simulink model "simp"  (R2012b)
settings: Solver=ode45  StartTime=0.0  StopTime=1000  FixedStep=0.01  RelTol=1e-3
values from neighbouring files (symbols this model uses):
  A43 = gama / Jp - (L * gama) / (Jp * beta)    (= 8.61159929701)    [para.m]    (also in test.m = 8.13653136531)
  B4 = (L / beta - 1) / Jp    (= -0.00439367311072)    [para.m]    (also in test.m = -0.00615006150062)
  f4 = 100    [para.m]
  gama1 = -4    [para.m]
  gama2 = -10000    [para.m]
  K2max = 100    [para.m]
  Kd0 = 2 * ksi * wn / B4    (= -3218.264)    [para.m]
  Kp0 = (wn ^ 2 + A43) / B4    (= -24720)    [para.m]
  ksi = 0.707    [para.m]
  Kthi0 = 1000    [para.m]
  p11 = ksi / wn + (wn ^ 2 + 1) / (4 * ksi)    (= 35.7849857143)    [para.m]
  p12 = 1 / (2 * wn ^ 2)    (= 0.005)    [para.m]
  p22 = (wn ^ 2 + 1) / (4 * ksi * wn ^ 3)    (= 0.0357142857143)    [para.m]
  wn = 10    [para.m]
settings Model: Creator=Administrator  LastModifiedBy=Administrator
settings DebuggingCC: MaxConsecutiveZCsMsg=warning

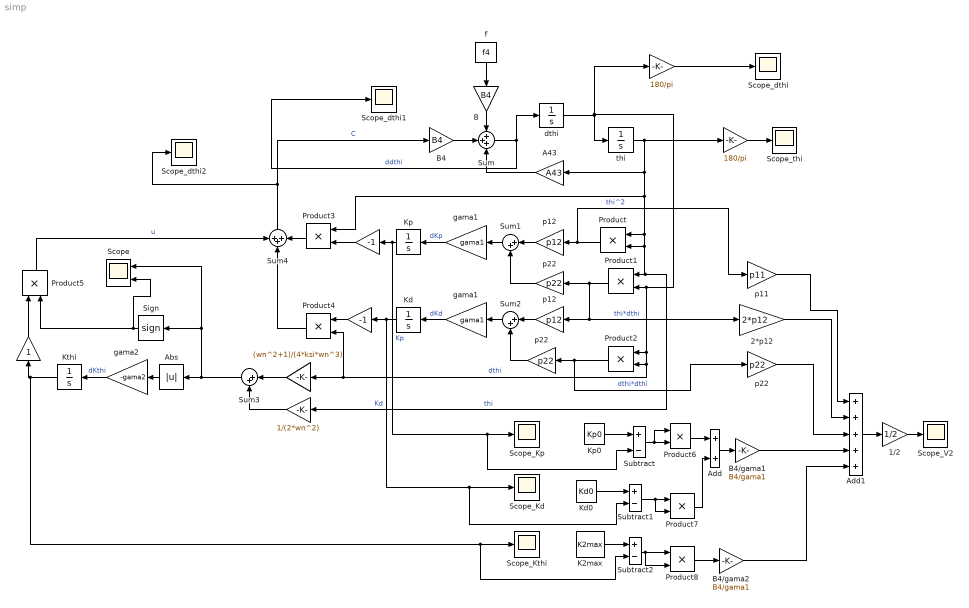
== system simp ==
  "    " : Gain  Gain=180/pi
  "         " : Gain  Gain=(wn^2+1)/(4*ksi*wn^3)
  "          " : Gain  Gain=1/(2*wn^2)
  "            " : Gain  Gain=-1
  "             " : Gain  Gain=180/pi
  "              " : Gain  Gain=-1
  "               " : Gain
  "  p11" : Gain  Gain=p11
  "  p12 " : Gain  Gain=p12
  " 2*p12" : Gain  Gain=2*p12
  1/2 : Gain  Gain=1/2
  A43 : Gain  Gain=A43
  Abs : Abs
  Add : Sum
  Add1 : Sum  Inputs=+++++
  B : Gain  Gain=B4
  B4 : Gain  Gain=B4
  B4/gama1 : Gain  Gain=B4/gama1
  B4/gama2 : Gain  Gain=B4/gama1
  K2max : Constant  Value=K2max
  Kd : Integrator  InitialCondition=Kd0
  Kd0 : Constant  Value=Kd0
  Kp : Integrator  InitialCondition=Kp0
  Kp0 : Constant  Value=Kp0
  Kthi : Integrator  InitialCondition=Kthi0
  Product{,1..8} (9 alike) : Product  RndMeth=Zero
  Scope : Scope  NumInputPorts=2
      settings: YMin=-5~-5  YMax=5~5  SaveName=ScopeData5
  Scope_Kd : Scope
      settings: SaveName=ScopeData3
  Scope_Kp : Scope
      settings: SaveName=ScopeData2
  Scope_Kthi : Scope
      settings: SaveName=ScopeData4
  Scope_V2 : Scope
      settings: SaveName=ScopeData6
  Scope_dthi : Scope
  Scope_dthi1 : Scope
      settings: SaveName=ScopeData7
  Scope_dthi2 : Scope
      settings: SaveName=ScopeData8
  Scope_thi : Scope
  Sign : Signum  ZeroCross=off
  Subtract : Sum  Inputs=+-
  Subtract1 : Sum  Inputs=+-
  Subtract2 : Sum  Inputs=+-
  Sum : Sum  Inputs=+++
  Sum1 : Sum  Inputs=|++
  Sum2 : Sum  Inputs=|++
  Sum3 : Sum  Inputs=|++
  Sum4 : Sum  Inputs=+++
  dthi : Integrator
  f : Constant  Value=f4
  gama1 : Gain  Gain=gama1
  "gama1      " : Gain  Gain=gama1
  gama2 : Gain  Gain=-gama2
  p12 : Gain  Gain=p12
  p22 : Gain  Gain=p22
  "p22 " : Gain  Gain=p22
  "p22  " : Gain  Gain=p22
  thi : Integrator  InitialCondition=15*pi/180
  wires:
  dthi/1 -> thi/1, Product4/2, "         "/1, Product2/2, Product2/1, Product1/2, "    "/1  "dthi"
  thi/1 -> "             "/1, Product1/1, "          "/1, Product/2, Product/1, Product3/1, A43/1  "thi"
  B4/1 -> Sum/2
  f/1 -> B/1
  A43/1 -> Sum/3
  Sum/1 -> dthi/1, Scope_dthi1/1  "ddthi"
  Product/1 -> "  p11"/1, p12/1  "thi^2"
  Product1/1 -> p22/1, " 2*p12"/1, "  p12 "/1  "thi*dthi"
  p12/1 -> Sum1/1
  p22/1 -> Sum1/2
  Product2/1 -> "p22 "/1, "p22  "/1  "dthi*dthi"
  "  p12 "/1 -> Sum2/1
  "p22  "/1 -> Sum2/2
  Sum1/1 -> "gama1      "/1
  Sum2/1 -> gama1/1
  "              "/1 -> Product3/2
  "            "/1 -> Product4/1
  "gama1      "/1 -> Kp/1  "dKp"
  gama1/1 -> Kd/1  "dKd"
  Product4/1 -> Sum4/2
  Product3/1 -> Sum4/3
  "         "/1 -> Sum3/1
  "          "/1 -> Sum3/2
  Sum3/1 -> Scope/1, Sign/1, Abs/1
  Abs/1 -> gama2/1
  gama2/1 -> Kthi/1  "dKthi"
  Kthi/1 -> Subtract2/2, Scope_Kthi/1, "               "/1
  "               "/1 -> Product5/1
  Sign/1 -> Scope/2, Product5/2
  Product5/1 -> Sum4/1  "u"
  Sum4/1 -> Scope_dthi2/1, B4/1  "C"
  B/1 -> Sum/1
  "    "/1 -> Scope_dthi/1
  "             "/1 -> Scope_thi/1
  Kd/1 -> Subtract1/2, Scope_Kd/1, "            "/1  "Kd"
  Kp/1 -> Subtract/2, Scope_Kp/1, "              "/1  "Kp"
  Kp0/1 -> Subtract/1
  Kd0/1 -> Subtract1/1
  Subtract/1 -> Product6/2, Product6/1
  Subtract1/1 -> Product7/2, Product7/1
  Product6/1 -> Add/1
  Product7/1 -> Add/2
  Add/1 -> B4/gama1/1
  K2max/1 -> Subtract2/1
  Subtract2/1 -> Product8/2, Product8/1
  Product8/1 -> B4/gama2/1
  "  p11"/1 -> Add1/1
  " 2*p12"/1 -> Add1/2
  "p22 "/1 -> Add1/3
  B4/gama1/1 -> Add1/4
  B4/gama2/1 -> Add1/5
  Add1/1 -> 1/2/1
  1/2/1 -> Scope_V2/1
